simulink library "Aritmetic_Blocks"  (Simulink 8.1)
settings: Solver=ode45  StartTime=0.0  StopTime=10.0  RelTol=1e-3
libraries: Common_Library x24, commutil2 x8
settings Model: Creator=uzivatel  LastModifiedBy=uzivatel

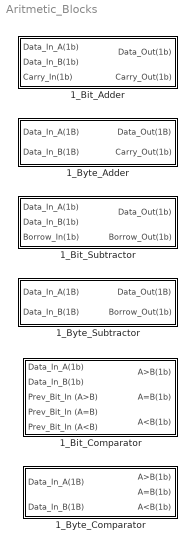
== system Aritmetic_Blocks ==
  1_Bit_Adder : Subsystem
  1_Bit_Comparator : Subsystem
  1_Bit_Subtractor : Subsystem
  1_Byte_Adder : Subsystem
  1_Byte_Comparator : Subsystem
  1_Byte_Subtractor : Subsystem

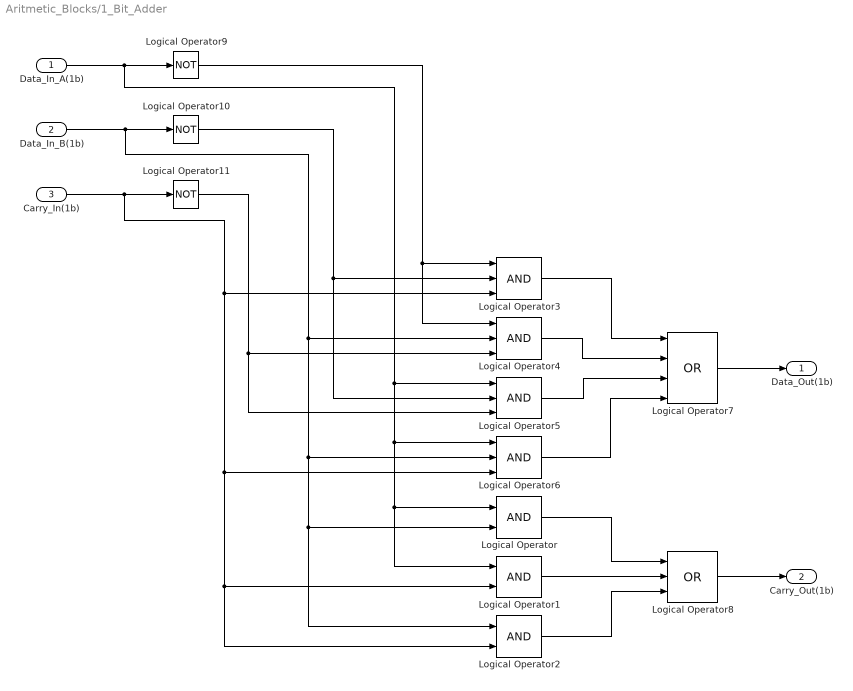
== system Aritmetic_Blocks/1_Bit_Adder ==
  Data_In_A(1b) : Inport
  Data_In_B(1b) : Inport  Port=2
  Carry_In(1b) : Inport  Port=3
  Logical Operator : Logic  IconShape=distinctive  AllPortsSameDT=off  OutDataTypeStr=boolean
  Logical Operator1 : Logic  IconShape=distinctive  AllPortsSameDT=off  OutDataTypeStr=boolean
  Logical Operator10 : Logic  Operator=NOT  Inputs=4  IconShape=distinctive  AllPortsSameDT=off  OutDataTypeStr=boolean
  Logical Operator11 : Logic  Operator=NOT  Inputs=4  IconShape=distinctive  AllPortsSameDT=off  OutDataTypeStr=boolean
  Logical Operator2 : Logic  IconShape=distinctive  AllPortsSameDT=off  OutDataTypeStr=boolean
  Logical Operator{3..6} (4 alike) : Logic  Inputs=3  IconShape=distinctive  AllPortsSameDT=off  OutDataTypeStr=boolean
  Logical Operator7 : Logic  Operator=OR  Inputs=4  IconShape=distinctive  AllPortsSameDT=off  OutDataTypeStr=boolean
  Logical Operator8 : Logic  Operator=OR  Inputs=3  IconShape=distinctive  AllPortsSameDT=off  OutDataTypeStr=boolean
  Logical Operator9 : Logic  Operator=NOT  Inputs=4  IconShape=distinctive  AllPortsSameDT=off  OutDataTypeStr=boolean
  Data_Out(1b) : Outport
  Carry_Out(1b) : Outport  Port=2
  wires:
  Logical Operator11/1 -> Logical Operator4/3, Logical Operator5/3
  Logical Operator10/1 -> Logical Operator3/2, Logical Operator5/2
  Logical Operator9/1 -> Logical Operator3/1, Logical Operator4/1
  Data_In_A(1b)/1 -> Logical Operator9/1, Logical Operator5/1, Logical Operator6/1, Logical Operator/1, Logical Operator1/1
  Data_In_B(1b)/1 -> Logical Operator10/1, Logical Operator4/2, Logical Operator6/2, Logical Operator/2, Logical Operator2/1
  Carry_In(1b)/1 -> Logical Operator11/1, Logical Operator3/3, Logical Operator6/3, Logical Operator1/2, Logical Operator2/2
  Logical Operator2/1 -> Logical Operator8/3
  Logical Operator1/1 -> Logical Operator8/2
  Logical Operator/1 -> Logical Operator8/1
  Logical Operator8/1 -> Carry_Out(1b)/1
  Logical Operator7/1 -> Data_Out(1b)/1
  Logical Operator6/1 -> Logical Operator7/4
  Logical Operator5/1 -> Logical Operator7/3
  Logical Operator4/1 -> Logical Operator7/2
  Logical Operator3/1 -> Logical Operator7/1

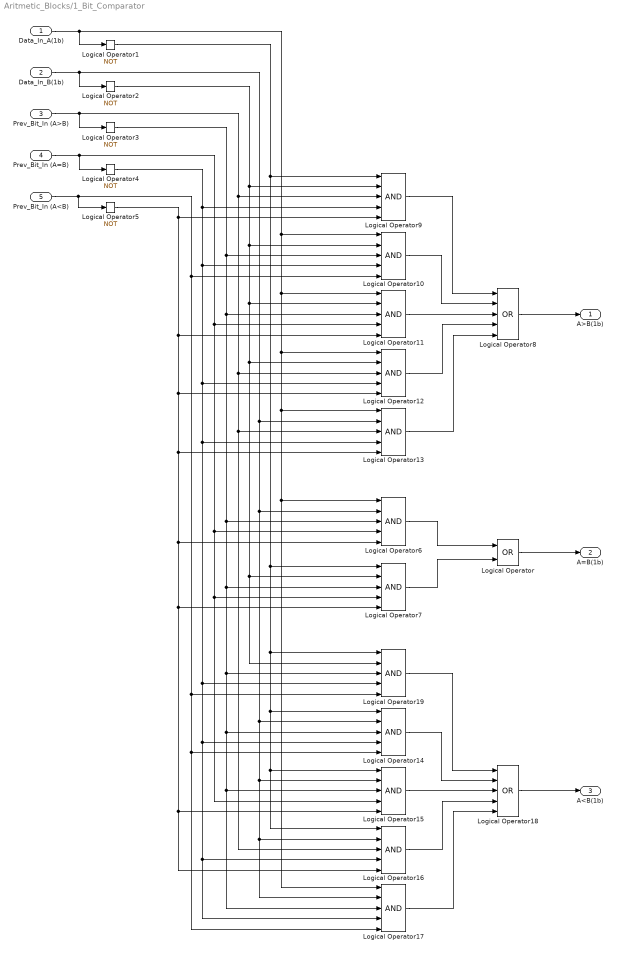
== system Aritmetic_Blocks/1_Bit_Comparator ==
  Data_In_A(1b) : Inport
  Data_In_B(1b) : Inport  Port=2
  Prev_Bit_In (A>B) : Inport  Port=3
  Prev_Bit_In (A=B) : Inport  Port=4
  Prev_Bit_In (A<B) : Inport  Port=5
  Logical Operator : Logic  Operator=OR  IconShape=distinctive  AllPortsSameDT=off  OutDataTypeStr=boolean
  Logical Operator{1..5} (5 alike) : Logic  Operator=NOT  IconShape=distinctive  AllPortsSameDT=off  OutDataTypeStr=boolean
  Logical Operator{6..7,9..17,19} (12 alike) : Logic  Inputs=5  IconShape=distinctive  AllPortsSameDT=off  OutDataTypeStr=boolean
  Logical Operator18 : Logic  Operator=OR  Inputs=5  IconShape=distinctive  AllPortsSameDT=off  OutDataTypeStr=boolean
  Logical Operator8 : Logic  Operator=OR  Inputs=5  IconShape=distinctive  AllPortsSameDT=off  OutDataTypeStr=boolean
  A>B(1b) : Outport
  A=B(1b) : Outport  Port=2
  A<B(1b) : Outport  Port=3
  wires:
  Logical Operator16/1 -> Logical Operator18/4
  Logical Operator17/1 -> Logical Operator18/5
  Logical Operator19/1 -> Logical Operator18/1
  Logical Operator15/1 -> Logical Operator18/3
  Logical Operator14/1 -> Logical Operator18/2
  Logical Operator4/1 -> Logical Operator9/4, Logical Operator10/4, Logical Operator12/4, Logical Operator13/4, Logical Operator19/4, Logical Operator14/4, Logical Operator17/4, Logical Operator16/4
  Data_In_A(1b)/1 -> Logical Operator10/1, Logical Operator11/1, Logical Operator12/1, Logical Operator13/1, Logical Operator6/1, Logical Operator17/1, Logical Operator1/1
  Logical Operator5/1 -> Logical Operator9/5, Logical Operator11/5, Logical Operator12/5, Logical Operator13/5, Logical Operator6/5, Logical Operator7/5, Logical Operator15/5, Logical Operator16/5
  Logical Operator18/1 -> A<B(1b)/1
  Logical Operator2/1 -> Logical Operator9/2, Logical Operator10/2, Logical Operator11/2, Logical Operator12/2, Logical Operator7/2, Logical Operator19/2
  Logical Operator1/1 -> Logical Operator9/1, Logical Operator7/1, Logical Operator19/1, Logical Operator14/1, Logical Operator15/1, Logical Operator16/1
  Logical Operator3/1 -> Logical Operator10/3, Logical Operator11/3, Logical Operator6/3, Logical Operator7/3, Logical Operator19/3, Logical Operator14/3, Logical Operator15/3, Logical Operator17/3
  Prev_Bit_In (A<B)/1 -> Logical Operator5/1, Logical Operator10/5, Logical Operator19/5, Logical Operator14/5, Logical Operator17/5
  Prev_Bit_In (A>B)/1 -> Logical Operator3/1, Logical Operator9/3, Logical Operator12/3, Logical Operator13/3, Logical Operator16/3
  Prev_Bit_In (A=B)/1 -> Logical Operator11/4, Logical Operator6/4, Logical Operator7/4, Logical Operator15/4, Logical Operator4/1
  Logical Operator6/1 -> Logical Operator/1
  Logical Operator7/1 -> Logical Operator/2
  Data_In_B(1b)/1 -> Logical Operator2/1, Logical Operator13/2, Logical Operator6/2, Logical Operator17/2, Logical Operator16/2, Logical Operator15/2, Logical Operator14/2
  Logical Operator/1 -> A=B(1b)/1
  Logical Operator8/1 -> A>B(1b)/1
  Logical Operator13/1 -> Logical Operator8/5
  Logical Operator11/1 -> Logical Operator8/3
  Logical Operator10/1 -> Logical Operator8/2
  Logical Operator12/1 -> Logical Operator8/4
  Logical Operator9/1 -> Logical Operator8/1

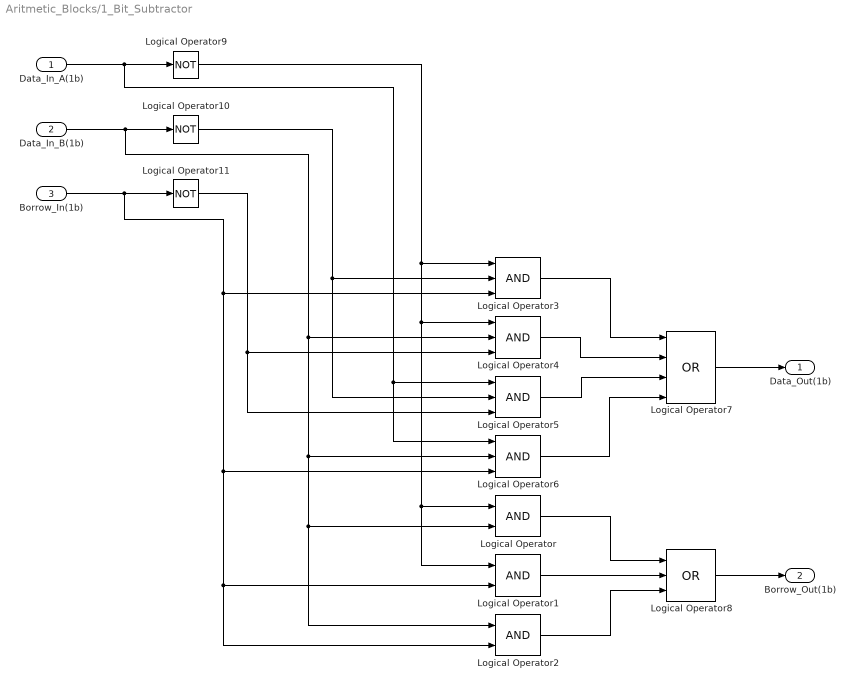
== system Aritmetic_Blocks/1_Bit_Subtractor ==
  Data_In_A(1b) : Inport
  Data_In_B(1b) : Inport  Port=2
  Borrow_In(1b) : Inport  Port=3
  Logical Operator : Logic  IconShape=distinctive  AllPortsSameDT=off  OutDataTypeStr=boolean
  Logical Operator1 : Logic  IconShape=distinctive  AllPortsSameDT=off  OutDataTypeStr=boolean
  Logical Operator10 : Logic  Operator=NOT  Inputs=4  IconShape=distinctive  AllPortsSameDT=off  OutDataTypeStr=boolean
  Logical Operator11 : Logic  Operator=NOT  Inputs=4  IconShape=distinctive  AllPortsSameDT=off  OutDataTypeStr=boolean
  Logical Operator2 : Logic  IconShape=distinctive  AllPortsSameDT=off  OutDataTypeStr=boolean
  Logical Operator{3..6} (4 alike) : Logic  Inputs=3  IconShape=distinctive  AllPortsSameDT=off  OutDataTypeStr=boolean
  Logical Operator7 : Logic  Operator=OR  Inputs=4  IconShape=distinctive  AllPortsSameDT=off  OutDataTypeStr=boolean
  Logical Operator8 : Logic  Operator=OR  Inputs=3  IconShape=distinctive  AllPortsSameDT=off  OutDataTypeStr=boolean
  Logical Operator9 : Logic  Operator=NOT  Inputs=4  IconShape=distinctive  AllPortsSameDT=off  OutDataTypeStr=boolean
  Data_Out(1b) : Outport
  Borrow_Out(1b) : Outport  Port=2
  wires:
  Logical Operator11/1 -> Logical Operator4/3, Logical Operator5/3
  Logical Operator10/1 -> Logical Operator3/2, Logical Operator5/2
  Logical Operator9/1 -> Logical Operator3/1, Logical Operator4/1, Logical Operator/1, Logical Operator1/1
  Data_In_A(1b)/1 -> Logical Operator9/1, Logical Operator5/1, Logical Operator6/1
  Data_In_B(1b)/1 -> Logical Operator10/1, Logical Operator4/2, Logical Operator6/2, Logical Operator/2, Logical Operator2/1
  Borrow_In(1b)/1 -> Logical Operator11/1, Logical Operator3/3, Logical Operator6/3, Logical Operator1/2, Logical Operator2/2
  Logical Operator2/1 -> Logical Operator8/3
  Logical Operator1/1 -> Logical Operator8/2
  Logical Operator/1 -> Logical Operator8/1
  Logical Operator8/1 -> Borrow_Out(1b)/1
  Logical Operator7/1 -> Data_Out(1b)/1
  Logical Operator6/1 -> Logical Operator7/4
  Logical Operator5/1 -> Logical Operator7/3
  Logical Operator4/1 -> Logical Operator7/2
  Logical Operator3/1 -> Logical Operator7/1

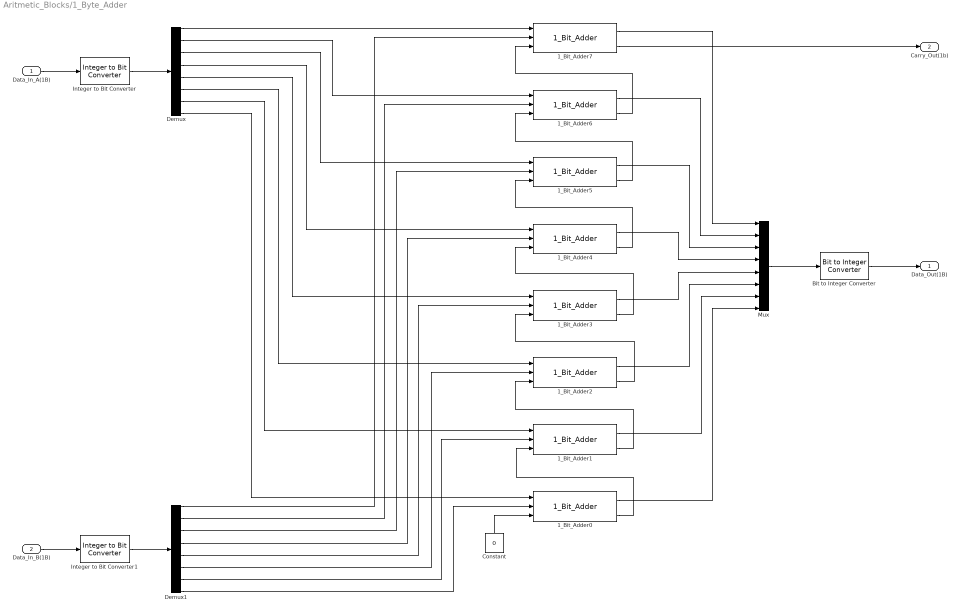
== system Aritmetic_Blocks/1_Byte_Adder ==
  Data_In_A(1B) : Inport
  Data_In_B(1B) : Inport  Port=2
  1_Bit_Adder{0..7} (8 alike) : Common_Library/Adders/1_Bit_Adder
  Bit to Integer Converter : commutil2/Bit to Integer Converter  nbits=8  bitOrder=MSB first  signedOutputValues=Unsigned  outDtype=uint8  outDtypeSigned=Inherit via internal rule
  Constant : Constant  Value=0
  Demux : Demux  Outputs=8
  Demux1 : Demux  Outputs=8
  Integer to Bit Converter : commutil2/Integer to Bit Converter  nbits=8  signedInputValues=Unsigned  bitOrder=MSB first  outDtype=uint8
  Integer to Bit Converter1 : commutil2/Integer to Bit Converter  nbits=8  signedInputValues=Unsigned  bitOrder=MSB first  outDtype=uint8
  Mux : Mux  Inputs=8
  Data_Out(1B) : Outport
  Carry_Out(1b) : Outport  Port=2
  wires:
  Bit to Integer Converter/1 -> Data_Out(1B)/1
  Mux/1 -> Bit to Integer Converter/1
  Integer to Bit Converter1/1 -> Demux1/1
  Data_In_B(1B)/1 -> Integer to Bit Converter1/1
  Integer to Bit Converter/1 -> Demux/1
  Data_In_A(1B)/1 -> Integer to Bit Converter/1
  1_Bit_Adder6/2 -> 1_Bit_Adder7/3
  1_Bit_Adder5/2 -> 1_Bit_Adder6/3
  1_Bit_Adder4/2 -> 1_Bit_Adder5/3
  1_Bit_Adder3/2 -> 1_Bit_Adder4/3
  1_Bit_Adder2/2 -> 1_Bit_Adder3/3
  1_Bit_Adder1/2 -> 1_Bit_Adder2/3
  1_Bit_Adder0/2 -> 1_Bit_Adder1/3
  1_Bit_Adder7/2 -> Carry_Out(1b)/1
  Constant/1 -> 1_Bit_Adder0/3
  Demux1/8 -> 1_Bit_Adder0/2
  Demux1/7 -> 1_Bit_Adder1/2
  Demux1/6 -> 1_Bit_Adder2/2
  Demux1/5 -> 1_Bit_Adder3/2
  Demux1/4 -> 1_Bit_Adder4/2
  Demux1/3 -> 1_Bit_Adder5/2
  Demux1/2 -> 1_Bit_Adder6/2
  Demux1/1 -> 1_Bit_Adder7/2
  Demux/8 -> 1_Bit_Adder0/1
  Demux/7 -> 1_Bit_Adder1/1
  Demux/6 -> 1_Bit_Adder2/1
  Demux/5 -> 1_Bit_Adder3/1
  Demux/4 -> 1_Bit_Adder4/1
  Demux/3 -> 1_Bit_Adder5/1
  Demux/2 -> 1_Bit_Adder6/1
  Demux/1 -> 1_Bit_Adder7/1
  1_Bit_Adder3/1 -> Mux/5
  1_Bit_Adder4/1 -> Mux/4
  1_Bit_Adder5/1 -> Mux/3
  1_Bit_Adder2/1 -> Mux/6
  1_Bit_Adder1/1 -> Mux/7
  1_Bit_Adder0/1 -> Mux/8
  1_Bit_Adder6/1 -> Mux/2
  1_Bit_Adder7/1 -> Mux/1

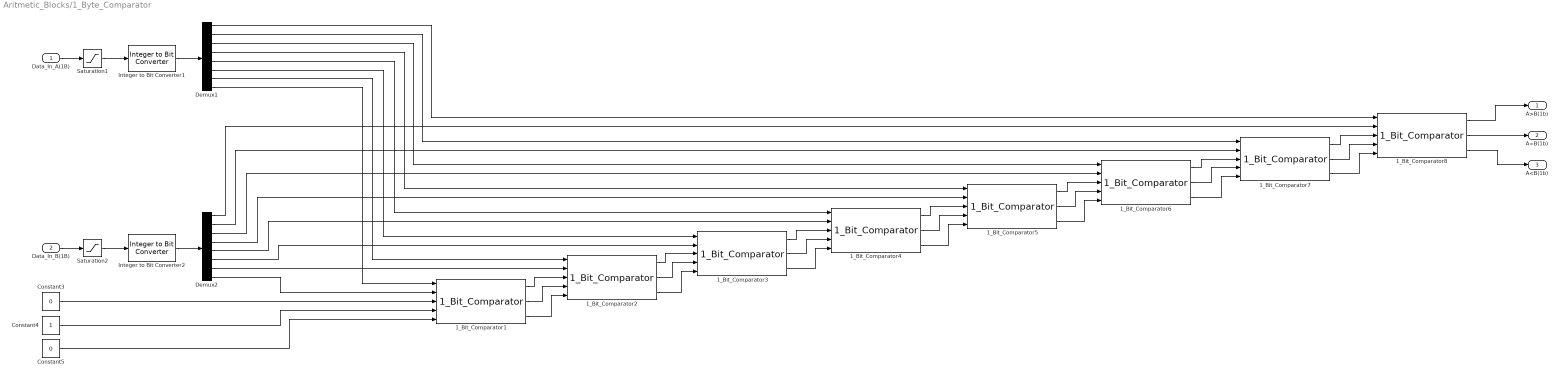
== system Aritmetic_Blocks/1_Byte_Comparator ==
  Data_In_A(1B) : Inport
  Data_In_B(1B) : Inport  Port=2
  1_Bit_Comparator{1..8} (8 alike) : Common_Library/Comparators/1_Bit_Comparator
  Constant3 : Constant  Value=0  OutDataTypeStr=int16
  Constant4 : Constant  OutDataTypeStr=int16
  Constant5 : Constant  Value=0  OutDataTypeStr=int16
  Demux1 : Demux  Outputs=8
  Demux2 : Demux  Outputs=8
  Integer to Bit Converter1 : commutil2/Integer to Bit Converter  nbits=8  signedInputValues=Unsigned  bitOrder=MSB first  outDtype=uint8
  Integer to Bit Converter2 : commutil2/Integer to Bit Converter  nbits=8  signedInputValues=Unsigned  bitOrder=MSB first  outDtype=uint8
  Saturation1 : Saturate  UpperLimit=255  LowerLimit=0
  Saturation2 : Saturate  UpperLimit=255  LowerLimit=0
  A>B(1b) : Outport
  A=B(1b) : Outport  Port=2
  A<B(1b) : Outport  Port=3
  wires:
  1_Bit_Comparator8/3 -> A<B(1b)/1
  1_Bit_Comparator8/1 -> A>B(1b)/1
  1_Bit_Comparator8/2 -> A=B(1b)/1
  Demux1/1 -> 1_Bit_Comparator8/1
  Demux1/2 -> 1_Bit_Comparator7/1
  Demux1/3 -> 1_Bit_Comparator6/1
  Demux1/4 -> 1_Bit_Comparator5/1
  Demux1/5 -> 1_Bit_Comparator4/1
  Demux1/6 -> 1_Bit_Comparator3/1
  Demux1/7 -> 1_Bit_Comparator2/1
  Data_In_A(1B)/1 -> Saturation1/1
  Saturation1/1 -> Integer to Bit Converter1/1
  Integer to Bit Converter1/1 -> Demux1/1
  Demux2/1 -> 1_Bit_Comparator8/2
  Demux2/2 -> 1_Bit_Comparator7/2
  Demux2/3 -> 1_Bit_Comparator6/2
  Demux2/4 -> 1_Bit_Comparator5/2
  Demux2/5 -> 1_Bit_Comparator4/2
  Demux2/6 -> 1_Bit_Comparator3/2
  Demux2/7 -> 1_Bit_Comparator2/2
  Data_In_B(1B)/1 -> Saturation2/1
  Saturation2/1 -> Integer to Bit Converter2/1
  Integer to Bit Converter2/1 -> Demux2/1
  1_Bit_Comparator7/3 -> 1_Bit_Comparator8/5
  1_Bit_Comparator7/2 -> 1_Bit_Comparator8/4
  1_Bit_Comparator7/1 -> 1_Bit_Comparator8/3
  1_Bit_Comparator6/3 -> 1_Bit_Comparator7/5
  1_Bit_Comparator6/2 -> 1_Bit_Comparator7/4
  1_Bit_Comparator6/1 -> 1_Bit_Comparator7/3
  1_Bit_Comparator5/3 -> 1_Bit_Comparator6/5
  1_Bit_Comparator5/2 -> 1_Bit_Comparator6/4
  1_Bit_Comparator5/1 -> 1_Bit_Comparator6/3
  1_Bit_Comparator4/3 -> 1_Bit_Comparator5/5
  1_Bit_Comparator4/2 -> 1_Bit_Comparator5/4
  1_Bit_Comparator4/1 -> 1_Bit_Comparator5/3
  1_Bit_Comparator3/3 -> 1_Bit_Comparator4/5
  1_Bit_Comparator3/2 -> 1_Bit_Comparator4/4
  1_Bit_Comparator3/1 -> 1_Bit_Comparator4/3
  1_Bit_Comparator2/3 -> 1_Bit_Comparator3/5
  1_Bit_Comparator2/1 -> 1_Bit_Comparator3/3
  1_Bit_Comparator2/2 -> 1_Bit_Comparator3/4
  Demux1/8 -> 1_Bit_Comparator1/1
  1_Bit_Comparator1/3 -> 1_Bit_Comparator2/5
  Demux2/8 -> 1_Bit_Comparator1/2
  Constant3/1 -> 1_Bit_Comparator1/3
  1_Bit_Comparator1/1 -> 1_Bit_Comparator2/3
  1_Bit_Comparator1/2 -> 1_Bit_Comparator2/4
  Constant5/1 -> 1_Bit_Comparator1/5
  Constant4/1 -> 1_Bit_Comparator1/4

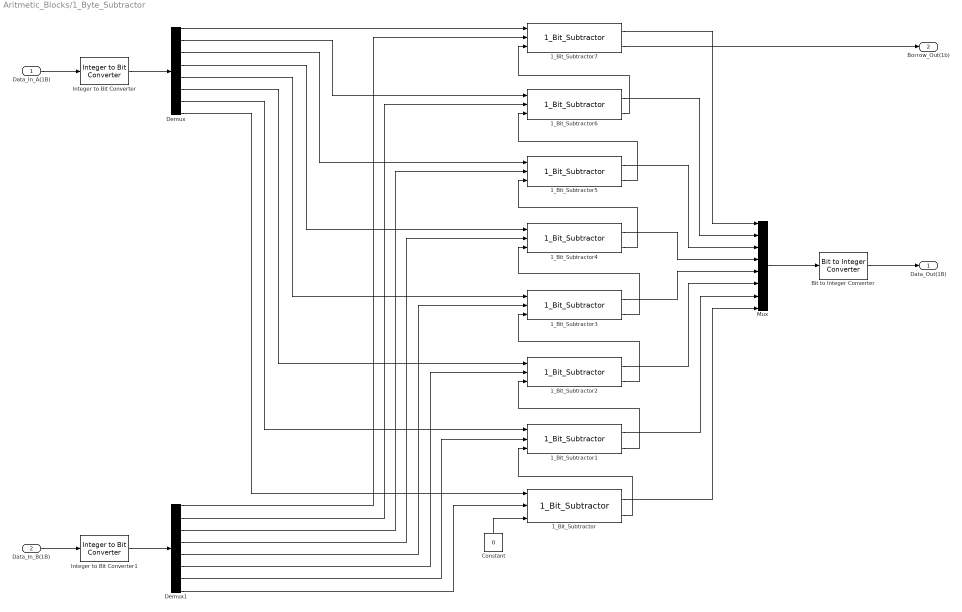
== system Aritmetic_Blocks/1_Byte_Subtractor ==
  Data_In_A(1B) : Inport
  Data_In_B(1B) : Inport  Port=2
  1_Bit_Subtractor{,1..7} (8 alike) : Common_Library/Subtractors/1_Bit_Subtractor
  Bit to Integer Converter : commutil2/Bit to Integer Converter  nbits=8  bitOrder=MSB first  signedOutputValues=Unsigned  outDtype=uint8  outDtypeSigned=Inherit via internal rule
  Constant : Constant  Value=0
  Demux : Demux  Outputs=8
  Demux1 : Demux  Outputs=8
  Integer to Bit Converter : commutil2/Integer to Bit Converter  nbits=8  signedInputValues=Unsigned  bitOrder=MSB first  outDtype=uint8
  Integer to Bit Converter1 : commutil2/Integer to Bit Converter  nbits=8  signedInputValues=Unsigned  bitOrder=MSB first  outDtype=uint8
  Mux : Mux  Inputs=8
  Data_Out(1B) : Outport
  Borrow_Out(1b) : Outport  Port=2
  wires:
  Bit to Integer Converter/1 -> Data_Out(1B)/1
  Mux/1 -> Bit to Integer Converter/1
  Integer to Bit Converter1/1 -> Demux1/1
  Data_In_B(1B)/1 -> Integer to Bit Converter1/1
  Integer to Bit Converter/1 -> Demux/1
  Data_In_A(1B)/1 -> Integer to Bit Converter/1
  1_Bit_Subtractor6/2 -> 1_Bit_Subtractor7/3
  1_Bit_Subtractor5/2 -> 1_Bit_Subtractor6/3
  1_Bit_Subtractor4/2 -> 1_Bit_Subtractor5/3
  1_Bit_Subtractor3/2 -> 1_Bit_Subtractor4/3
  1_Bit_Subtractor2/2 -> 1_Bit_Subtractor3/3
  1_Bit_Subtractor1/2 -> 1_Bit_Subtractor2/3
  1_Bit_Subtractor/2 -> 1_Bit_Subtractor1/3
  1_Bit_Subtractor7/2 -> Borrow_Out(1b)/1
  Constant/1 -> 1_Bit_Subtractor/3
  Demux1/8 -> 1_Bit_Subtractor/2
  Demux1/7 -> 1_Bit_Subtractor1/2
  Demux1/6 -> 1_Bit_Subtractor2/2
  Demux1/5 -> 1_Bit_Subtractor3/2
  Demux1/4 -> 1_Bit_Subtractor4/2
  Demux1/3 -> 1_Bit_Subtractor5/2
  Demux1/2 -> 1_Bit_Subtractor6/2
  Demux1/1 -> 1_Bit_Subtractor7/2
  Demux/8 -> 1_Bit_Subtractor/1
  Demux/7 -> 1_Bit_Subtractor1/1
  Demux/6 -> 1_Bit_Subtractor2/1
  Demux/5 -> 1_Bit_Subtractor3/1
  Demux/4 -> 1_Bit_Subtractor4/1
  Demux/3 -> 1_Bit_Subtractor5/1
  Demux/2 -> 1_Bit_Subtractor6/1
  Demux/1 -> 1_Bit_Subtractor7/1
  1_Bit_Subtractor3/1 -> Mux/5
  1_Bit_Subtractor4/1 -> Mux/4
  1_Bit_Subtractor5/1 -> Mux/3
  1_Bit_Subtractor2/1 -> Mux/6
  1_Bit_Subtractor1/1 -> Mux/7
  1_Bit_Subtractor/1 -> Mux/8
  1_Bit_Subtractor6/1 -> Mux/2
  1_Bit_Subtractor7/1 -> Mux/1
